simulink model "Active_Suspension_LQR"  (Simulink 10.1)
settings: Solver=ode3  StartTime=0.0  StopTime=50  FixedStep=0.005  RelTol=1e-3  EnableMultiTasking=on
undefined symbols (not defined in the file): A, B, C, D, G, K
settings Model: Creator=tongji_HEV  LastModifiedBy=35668
settings DataIOCC: LimitDataPoints=on  SignalLoggingSaveFormat=ModelDataLogs
settings OptimizationCC: ExpressionDepthLimit=2147483647
settings DebuggingCC: SolverPrmCheckMsg=warning  FcnCallInpInsideContextMsg=warning  StateNameClashWarn=warning

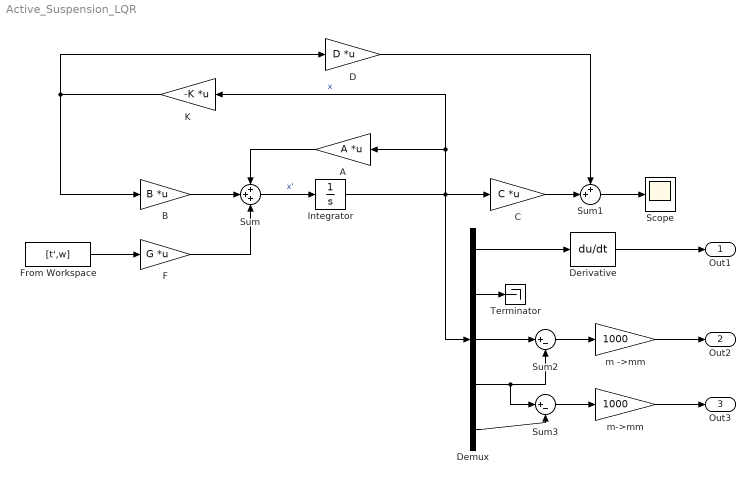
== system Active_Suspension_LQR ==
  A : Gain  Gain=A  Multiplication=Matrix(K*u)
  B : Gain  Gain=B  Multiplication=Matrix(K*u)
  C : Gain  Gain=C  Multiplication=Matrix(K*u)
  D : Gain  Gain=D  Multiplication=Matrix(K*u)
  Demux : Demux  Outputs=5
  Derivative : Derivative
  F : Gain  Gain=G  Multiplication=Matrix(K*u)
  From Workspace : FromWorkspace  VariableName=[t',w]  SampleTime=0.005
  Integrator : Integrator
  K : Gain  Gain=-K  Multiplication=Matrix(K*u)
  Scope : Scope
  Sum : Sum  Inputs=+++
  Sum1 : Sum  Inputs=++|
  Sum2 : Sum  Inputs=|+-
  Sum3 : Sum  Inputs=|+-
  Terminator : Terminator
  m ->mm : Gain  Gain=1000
  m->mm : Gain  Gain=1000
  Out1 : Outport
  Out2 : Outport  Port=2
  Out3 : Outport  Port=3
  wires:
  Integrator/1 -> A/1, K/1, C/1, Demux/1  "x"
  Sum/1 -> Integrator/1  "x'"
  D/1 -> Sum1/1
  C/1 -> Sum1/2
  Sum1/1 -> Scope/1
  A/1 -> Sum/1
  B/1 -> Sum/2
  F/1 -> Sum/3
  From Workspace/1 -> F/1
  K/1 -> B/1, D/1
  Demux/1 -> Derivative/1
  Demux/4 -> Sum2/2, Sum3/1
  Demux/5 -> Sum3/2
  Derivative/1 -> Out1/1
  Sum2/1 -> m ->mm/1
  Sum3/1 -> m->mm/1
  Demux/2 -> Terminator/1
  m->mm/1 -> Out3/1
  Demux/3 -> Sum2/1
  m ->mm/1 -> Out2/1
